simulink model "stability_analysis"  (R2022b)
settings: Solver=VariableStepAuto  StartTime=0.0  StopTime=10  RelTol=1e-3
undefined symbols (not defined in the file): A_dynamic_matrix, B_dynamic_matrix
libraries: Solver_SF x1
settings Model: Creator=Miakho  LastModifiedBy=Miakho

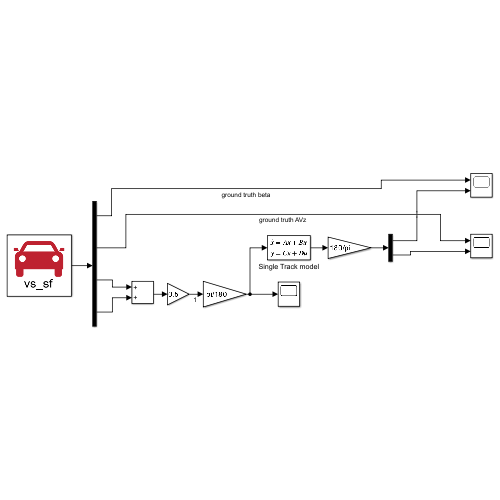
[thumbnail: Simulink's stored preview of the top-level diagram]
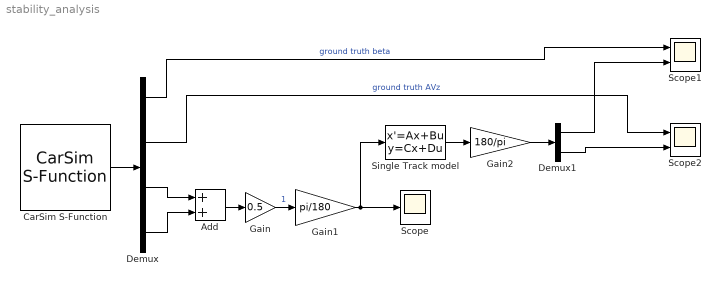
== system stability_analysis ==
  Add : Sum
  CarSim S-Function : Solver_SF/CarSim S-Function  Priority=1  SIMFILE=simfile.sim  Run_RTs=off  vs_state_ind=Run  StopMode_ind=Vehicle Model
  Demux : Demux
  Demux1 : Demux  Outputs=2
  Gain : Gain  Gain=0.5
  Gain1 : Gain  Gain=pi/180
  Gain2 : Gain  Gain=180/pi
  Scope : Scope
  Scope1 : Scope  NumInputPorts=2
  Scope2 : Scope  NumInputPorts=2
  Single Track model : StateSpace  A=A_dynamic_matrix  B=B_dynamic_matrix  C=eye(2)  D=zeros(2,1)  InitialCondition=0
  wires:
  CarSim S-Function/1 -> Demux/1
  Demux/3 -> Add/1
  Demux/4 -> Add/2
  Add/1 -> Gain/1
  Gain/1 -> Gain1/1  "1"
  Single Track model/1 -> Gain2/1
  Demux/1 -> Scope1/1  "ground truth beta"
  Demux/2 -> Scope2/1  "ground truth AVz"
  Demux1/2 -> Scope2/2
  Demux1/1 -> Scope1/2
  Gain1/1 -> Single Track model/1, Scope/1
  Gain2/1 -> Demux1/1
